simulink library "Miscellaneous"  (R2023a)
settings: Solver=ode45  StartTime=0.0  StopTime=10.0  RelTol=1e-3  EnableMultiTasking=on
libraries: simulink x4
(part 2 of 2)

== matlab function Miscellaneous/Merge2_Simulated/Merge_Simulated1 ==
  data: DataOut output Bus: BUS_UINT16_T; Data_1 input Bus: BUS_UINT16_T; Data_0 input Bus: BUS_UINT16_T
function DataOut = Or2(Data_1, Data_0)
    DataOut.b15 = Data_1.b15 || Data_0.b15;
    DataOut.b14 = Data_1.b14 || Data_0.b14;
    DataOut.b13 = Data_1.b13 || Data_0.b13;
    DataOut.b12 = Data_1.b12 || Data_0.b12;
    DataOut.b11 = Data_1.b11 || Data_0.b11;
    DataOut.b10 = Data_1.b10 || Data_0.b10;
    DataOut.b09 = Data_1.b09 || Data_0.b09;
    DataOut.b08 = Data_1.b08 || Data_0.b08;
    DataOut.b07 = Data_1.b07 || Data_0.b07;
    DataOut.b06 = Data_1.b06 || Data_0.b06;
    DataOut.b05 = Data_1.b05 || Data_0.b05;
    DataOut.b04 = Data_1.b04 || Data_0.b04;
    DataOut.b03 = Data_1.b03 || Data_0.b03;
    DataOut.b02 = Data_1.b02 || Data_0.b02;
    DataOut.b01 = Data_1.b01 || Data_0.b01;
    DataOut.b00 = Data_1.b00 || Data_0.b00;
end

== matlab function Miscellaneous/Merge16_Simulated ==
  data: Data_15 input Bus: BUS_UINT16_T; Data_14 input Bus: BUS_UINT16_T; Data_13 input Bus: BUS_UINT16_T size=1; Data_12 input Bus: BUS_UINT16_T; Data_11 input Bus: BUS_UINT16_T; Data_10 input Bus: BUS_UINT16_T; Data_09 input Bus: BUS_UINT16_T; Data_08 input Bus: BUS_UINT16_T; Data_07 input Bus: BUS_UINT16_T; Data_06 input Bus: BUS_UINT16_T; Data_05 input Bus: BUS_UINT16_T; Data_04 input Bus: BUS_UINT16_T; DataOut output Bus: BUS_UINT16_T; Data_03 input Bus: BUS_UINT16_T; Data_02 input Bus: BUS_UINT16_T; Data_01 input Bus: BUS_UINT16_T; Data_00 input Bus: BUS_UINT16_T
function DataOut = Or16(Data_15, Data_14, Data_13, Data_12, Data_11, Data_10, Data_09, Data_08, Data_07, Data_06, Data_05, Data_04, Data_03, Data_02, Data_01, Data_00)
    DataOut.b15 = Data_15.b15 || Data_14.b15 || Data_13.b15 || Data_12.b15 || Data_11.b15 || Data_10.b15 || Data_09.b15 || Data_08.b15 || Data_07.b15 || Data_06.b15 || Data_05.b15 || Data_04.b15 || Data_03.b15 || Data_02.b15 || Data_01.b15 || Data_00.b15;
    DataOut.b14 = Data_15.b14 || Data_14.b14 || Data_13.b14 || Data_12.b14 || Data_11.b14 || Data_10.b14 || Data_09.b14 || Data_08.b14 || Data_07.b14 || Data_06.b14 || Data_05.b14 || Data_04.b14 || Data_03.b14 || Data_02.b14 || Data_01.b14 || Data_00.b14;
    DataOut.b13 = Data_15.b13 || Data_14.b13 || Data_13.b13 || Data_12.b13 || Data_11.b13 || Data_10.b13 || Data_09.b13 || Data_08.b13 || Data_07.b13 || Data_06.b13 || Data_05.b13 || Data_04.b13 || Data_03.b13 || Data_02.b13 || Data_01.b13 || Data_00.b13;
    DataOut.b12 = Data_15.b12 || Data_14.b12 || Data_13.b12 || Data_12.b12 || Data_11.b12 || Data_10.b12 || Data_09.b12 || Data_08.b12 || Data_07.b12 || Data_06.b12 || Data_05.b12 || Data_04.b12 || Data_03.b12 || Data_02.b12 || Data_01.b12 || Data_00.b12;
    DataOut.b11 = Data_15.b11 || Data_14.b11 || Data_13.b11 || Data_12.b11 || Data_11.b11 || Data_10.b11 || Data_09.b11 || Data_08.b11 || Data_07.b11 || Data_06.b11 || Data_05.b11 || Data_04.b11 || Data_03.b11 || Data_02.b11 || Data_01.b11 || Data_00.b11;
    DataOut.b10 = Data_15.b10 || Data_14.b10 || Data_13.b10 || Data_12.b10 || Data_11.b10 || Data_10.b10 || Data_09.b10 || Data_08.b10 || Data_07.b10 || Data_06.b10 || Data_05.b10 || Data_04.b10 || Data_03.b10 || Data_02.b10 || Data_01.b10 || Data_00.b10;
    DataOut.b09 = Data_15.b09 || Data_14.b09 || Data_13.b09 || Data_12.b09 || Data_11.b09 || Data_10.b09 || Data_09.b09 || Data_08.b09 || Data_07.b09 || Data_06.b09 || Data_05.b09 || Data_04.b09 || Data_03.b09 || Data_02.b09 || Data_01.b09 || Data_00.b09;
    DataOut.b08 = Data_15.b08 || Data_14.b08 || Data_13.b08 || Data_12.b08 || Data_11.b08 || Data_10.b08 || Data_09.b08 || Data_08.b08 || Data_07.b08 || Data_06.b08 || Data_05.b08 || Data_04.b08 || Data_03.b08 || Data_02.b08 || Data_01.b08 || Data_00.b08;
    DataOut.b07 = Data_15.b07 || Data_14.b07 || Data_13.b07 || Data_12.b07 || Data_11.b07 || Data_10.b07 || Data_09.b07 || Data_08.b07 || Data_07.b07 || Data_06.b07 || Data_05.b07 || Data_04.b07 || Data_03.b07 || Data_02.b07 || Data_01.b07 || Data_00.b07;
    DataOut.b06 = Data_15.b06 || Data_14.b06 || Data_13.b06 || Data_12.b06 || Data_11.b06 || Data_10.b06 || Data_09.b06 || Data_08.b06 || Data_07.b06 || Data_06.b06 || Data_05.b06 || Data_04.b06 || Data_03.b06 || Data_02.b06 || Data_01.b06 || Data_00.b06;
    DataOut.b05 = Data_15.b05 || Data_14.b05 || Data_13.b05 || Data_12.b05 || Data_11.b05 || Data_10.b05 || Data_09.b05 || Data_08.b05 || Data_07.b05 || Data_06.b05 || Data_05.b05 || Data_04.b05 || Data_03.b05 || Data_02.b05 || Data_01.b05 || Data_00.b05;
    DataOut.b04 = Data_15.b04 || Data_14.b04 || Data_13.b04 || Data_12.b04 || Data_11.b04 || Data_10.b04 || Data_09.b04 || Data_08.b04 || Data_07.b04 || Data_06.b04 || Data_05.b04 || Data_04.b04 || Data_03.b04 || Data_02.b04 || Data_01.b04 || Data_00.b04;
    DataOut.b03 = Data_15.b03 || Data_14.b03 || Data_13.b03 || Data_12.b03 || Data_11.b03 || Data_10.b03 || Data_09.b03 || Data_08.b03 || Data_07.b03 || Data_06.b03 || Data_05.b03 || Data_04.b03 || Data_03.b03 || Data_02.b03 || Data_01.b03 || Data_00.b03;
    DataOut.b02 = Data_15.b02 || Data_14.b02 || Data_13.b02 || Data_12.b02 || Data_11.b02 || Data_10.b02 || Data_09.b02 || Data_08.b02 || Data_07.b02 || Data_06.b02 || Data_05.b02 || Data_04.b02 || Data_03.b02 || Data_02.b02 || Data_01.b02 || Data_00.b02;
    DataOut.b01 = Data_15.b01 || Data_14.b01 || Data_13.b01 || Data_12.b01 || Data_11.b01 || Data_10.b01 || Data_09.b01 || Data_08.b01 || Data_07.b01 || Data_06.b01 || Data_05.b01 || Data_04.b01 || Data_03.b01 || Data_02.b01 || Data_01.b01 || Data_00.b01;
    DataOut.b00 = Data_15.b00 || Data_14.b00 || Data_13.b00 || Data_12.b00 || Data_11.b00 || Data_10.b00 || Data_09.b00 || Data_08.b00 || Data_07.b00 || Data_06.b00 || Data_05.b00 || Data_04.b00 || Data_03.b00 || Data_02.b00 || Data_01.b00 || Data_00.b00;
end

== matlab function Miscellaneous/Merge8_Simulated ==
  data: Data_07 input Bus: BUS_UINT16_T; Data_06 input Bus: BUS_UINT16_T; Data_05 input Bus: BUS_UINT16_T; Data_04 input Bus: BUS_UINT16_T; DataOut output Bus: BUS_UINT16_T; Data_03 input Bus: BUS_UINT16_T; Data_02 input Bus: BUS_UINT16_T; Data_01 input Bus: BUS_UINT16_T; Data_00 input Bus: BUS_UINT16_T
function DataOut = Or8(Data_07, Data_06, Data_05, Data_04, Data_03, Data_02, Data_01, Data_00)
    DataOut.b15 = Data_07.b15 || Data_06.b15 || Data_05.b15 || Data_04.b15 || Data_03.b15 || Data_02.b15 || Data_01.b15 || Data_00.b15;
    DataOut.b14 = Data_07.b14 || Data_06.b14 || Data_05.b14 || Data_04.b14 || Data_03.b14 || Data_02.b14 || Data_01.b14 || Data_00.b14;
    DataOut.b13 = Data_07.b13 || Data_06.b13 || Data_05.b13 || Data_04.b13 || Data_03.b13 || Data_02.b13 || Data_01.b13 || Data_00.b13;
    DataOut.b12 = Data_07.b12 || Data_06.b12 || Data_05.b12 || Data_04.b12 || Data_03.b12 || Data_02.b12 || Data_01.b12 || Data_00.b12;
    DataOut.b11 = Data_07.b11 || Data_06.b11 || Data_05.b11 || Data_04.b11 || Data_03.b11 || Data_02.b11 || Data_01.b11 || Data_00.b11;
    DataOut.b10 = Data_07.b10 || Data_06.b10 || Data_05.b10 || Data_04.b10 || Data_03.b10 || Data_02.b10 || Data_01.b10 || Data_00.b10;
    DataOut.b09 = Data_07.b09 || Data_06.b09 || Data_05.b09 || Data_04.b09 || Data_03.b09 || Data_02.b09 || Data_01.b09 || Data_00.b09;
    DataOut.b08 = Data_07.b08 || Data_06.b08 || Data_05.b08 || Data_04.b08 || Data_03.b08 || Data_02.b08 || Data_01.b08 || Data_00.b08;
    DataOut.b07 = Data_07.b07 || Data_06.b07 || Data_05.b07 || Data_04.b07 || Data_03.b07 || Data_02.b07 || Data_01.b07 || Data_00.b07;
    DataOut.b06 = Data_07.b06 || Data_06.b06 || Data_05.b06 || Data_04.b06 || Data_03.b06 || Data_02.b06 || Data_01.b06 || Data_00.b06;
    DataOut.b05 = Data_07.b05 || Data_06.b05 || Data_05.b05 || Data_04.b05 || Data_03.b05 || Data_02.b05 || Data_01.b05 || Data_00.b05;
    DataOut.b04 = Data_07.b04 || Data_06.b04 || Data_05.b04 || Data_04.b04 || Data_03.b04 || Data_02.b04 || Data_01.b04 || Data_00.b04;
    DataOut.b03 = Data_07.b03 || Data_06.b03 || Data_05.b03 || Data_04.b03 || Data_03.b03 || Data_02.b03 || Data_01.b03 || Data_00.b03;
    DataOut.b02 = Data_07.b02 || Data_06.b02 || Data_05.b02 || Data_04.b02 || Data_03.b02 || Data_02.b02 || Data_01.b02 || Data_00.b02;
    DataOut.b01 = Data_07.b01 || Data_06.b01 || Data_05.b01 || Data_04.b01 || Data_03.b01 || Data_02.b01 || Data_01.b01 || Data_00.b01;
    DataOut.b00 = Data_07.b00 || Data_06.b00 || Data_05.b00 || Data_04.b00 || Data_03.b00 || Data_02.b00 || Data_01.b00 || Data_00.b00;
end

== matlab function Miscellaneous/Merge32_Simulated ==
  data: Data_31 input Bus: BUS_UINT16_T; Data_30 input Bus: BUS_UINT16_T; Data_29 input Bus: BUS_UINT16_T; Data_28 input Bus: BUS_UINT16_T; Data_27 input Bus: BUS_UINT16_T; Data_26 input Bus: BUS_UINT16_T; Data_25 input Bus: BUS_UINT16_T; Data_24 input Bus: BUS_UINT16_T; Data_23 input Bus: BUS_UINT16_T; Data_22 input Bus: BUS_UINT16_T; Data_21 input Bus: BUS_UINT16_T; Data_20 input Bus: BUS_UINT16_T; Data_19 input Bus: BUS_UINT16_T; Data_18 input Bus: BUS_UINT16_T; Data_17 input Bus: BUS_UINT16_T; Data_16 input Bus: BUS_UINT16_T; Data_15 input Bus: BUS_UINT16_T; Data_14 input Bus: BUS_UINT16_T; Data_13 input Bus: BUS_UINT16_T size=1; Data_12 input Bus: BUS_UINT16_T; Data_11 input Bus: BUS_UINT16_T; Data_10 input Bus: BUS_UINT16_T; Data_09 input Bus: BUS_UINT16_T; Data_08 input Bus: BUS_UINT16_T; Data_07 input Bus: BUS_UINT16_T; Data_06 input Bus: BUS_UINT16_T; Data_05 input Bus: BUS_UINT16_T; Data_04 input Bus: BUS_UINT16_T; DataOut output Bus: BUS_UINT16_T; Data_03 input Bus: BUS_UINT16_T; Data_02 input Bus: BUS_UINT16_T; Data_01 input Bus: BUS_UINT16_T; Data_00 input Bus: BUS_UINT16_T
function DataOut = Or32(Data_31, Data_30, Data_29, Data_28, Data_27, Data_26, Data_25, Data_24, Data_23, Data_22, Data_21, Data_20, Data_19, Data_18, Data_17, Data_16, Data_15, Data_14, Data_13, Data_12, Data_11, Data_10, Data_09, Data_08, Data_07, Data_06, Data_05, Data_04, Data_03, Data_02, Data_01, Data_00)
    DataOut.b15 = Data_31.b15 || Data_30.b15 || Data_29.b15 || Data_28.b15 || Data_27.b15 || Data_26.b15 || Data_25.b15 || Data_24.b15 || Data_23.b15 || Data_22.b15 || Data_21.b15 || Data_20.b15 || Data_19.b15 || Data_18.b15 || Data_17.b15 || Data_16.b15 || Data_15.b15 || Data_14.b15 || Data_13.b15 || Data_12.b15 || Data_11.b15 || Data_10.b15 || Data_09.b15 || Data_08.b15 || Data_07.b15 || Data_06.b15 || Data_05.b15 || Data_04.b15 || Data_03.b15 || Data_02.b15 || Data_01.b15 || Data_00.b15;
    DataOut.b14 = Data_31.b14 || Data_30.b14 || Data_29.b14 || Data_28.b14 || Data_27.b14 || Data_26.b14 || Data_25.b14 || Data_24.b14 || Data_23.b14 || Data_22.b14 || Data_21.b14 || Data_20.b14 || Data_19.b14 || Data_18.b14 || Data_17.b14 || Data_16.b14 || Data_15.b14 || Data_14.b14 || Data_13.b14 || Data_12.b14 || Data_11.b14 || Data_10.b14 || Data_09.b14 || Data_08.b14 || Data_07.b14 || Data_06.b14 || Data_05.b14 || Data_04.b14 || Data_03.b14 || Data_02.b14 || Data_01.b14 || Data_00.b14;
    DataOut.b13 = Data_31.b13 || Data_30.b13 || Data_29.b13 || Data_28.b13 || Data_27.b13 || Data_26.b13 || Data_25.b13 || Data_24.b13 || Data_23.b13 || Data_22.b13 || Data_21.b13 || Data_20.b13 || Data_19.b13 || Data_18.b13 || Data_17.b13 || Data_16.b13 || Data_15.b13 || Data_14.b13 || Data_13.b13 || Data_12.b13 || Data_11.b13 || Data_10.b13 || Data_09.b13 || Data_08.b13 || Data_07.b13 || Data_06.b13 || Data_05.b13 || Data_04.b13 || Data_03.b13 || Data_02.b13 || Data_01.b13 || Data_00.b13;
    DataOut.b12 = Data_31.b12 || Data_30.b12 || Data_29.b12 || Data_28.b12 || Data_27.b12 || Data_26.b12 || Data_25.b12 || Data_24.b12 || Data_23.b12 || Data_22.b12 || Data_21.b12 || Data_20.b12 || Data_19.b12 || Data_18.b12 || Data_17.b12 || Data_16.b12 || Data_15.b12 || Data_14.b12 || Data_13.b12 || Data_12.b12 || Data_11.b12 || Data_10.b12 || Data_09.b12 || Data_08.b12 || Data_07.b12 || Data_06.b12 || Data_05.b12 || Data_04.b12 || Data_03.b12 || Data_02.b12 || Data_01.b12 || Data_00.b12;
    DataOut.b11 = Data_31.b11 || Data_30.b11 || Data_29.b11 || Data_28.b11 || Data_27.b11 || Data_26.b11 || Data_25.b11 || Data_24.b11 || Data_23.b11 || Data_22.b11 || Data_21.b11 || Data_20.b11 || Data_19.b11 || Data_18.b11 || Data_17.b11 || Data_16.b11 || Data_15.b11 || Data_14.b11 || Data_13.b11 || Data_12.b11 || Data_11.b11 || Data_10.b11 || Data_09.b11 || Data_08.b11 || Data_07.b11 || Data_06.b11 || Data_05.b11 || Data_04.b11 || Data_03.b11 || Data_02.b11 || Data_01.b11 || Data_00.b11;
    DataOut.b10 = Data_31.b10 || Data_30.b10 || Data_29.b10 || Data_28.b10 || Data_27.b10 || Data_26.b10 || Data_25.b10 || Data_24.b10 || Data_23.b10 || Data_22.b10 || Data_21.b10 || Data_20.b10 || Data_19.b10 || Data_18.b10 || Data_17.b10 || Data_16.b10 || Data_15.b10 || Data_14.b10 || Data_13.b10 || Data_12.b10 || Data_11.b10 || Data_10.b10 || Data_09.b10 || Data_08.b10 || Data_07.b10 || Data_06.b10 || Data_05.b10 || Data_04.b10 || Data_03.b10 || Data_02.b10 || Data_01.b10 || Data_00.b10;
    DataOut.b09 = Data_31.b09 || Data_30.b09 || Data_29.b09 || Data_28.b09 || Data_27.b09 || Data_26.b09 || Data_25.b09 || Data_24.b09 || Data_23.b09 || Data_22.b09 || Data_21.b09 || Data_20.b09 || Data_19.b09 || Data_18.b09 || Data_17.b09 || Data_16.b09 || Data_15.b09 || Data_14.b09 || Data_13.b09 || Data_12.b09 || Data_11.b09 || Data_10.b09 || Data_09.b09 || Data_08.b09 || Data_07.b09 || Data_06.b09 || Data_05.b09 || Data_04.b09 || Data_03.b09 || Data_02.b09 || Data_01.b09 || Data_00.b09;
    DataOut.b08 = Data_31.b08 || Data_30.b08 || Data_29.b08 || Data_28.b08 || Data_27.b08 || Data_26.b08 || Data_25.b08 || Data_24.b08 || Data_23.b08 || Data_22.b08 || Data_21.b08 || Data_20.b08 || Data_19.b08 || Data_18.b08 || Data_17.b08 || Data_16.b08 || Data_15.b08 || Data_14.b08 || Data_13.b08 || Data_12.b08 || Data_11.b08 || Data_10.b08 || Data_09.b08 || Data_08.b08 || Data_07.b08 || Data_06.b08 || Data_05.b08 || Data_04.b08 || Data_03.b08 || Data_02.b08 || Data_01.b08 || Data_00.b08;
    DataOut.b07 = Data_31.b07 || Data_30.b07 || Data_29.b07 || Data_28.b07 || Data_27.b07 || Data_26.b07 || Data_25.b07 || Data_24.b07 || Data_23.b07 || Data_22.b07 || Data_21.b07 || Data_20.b07 || Data_19.b07 || Data_18.b07 || Data_17.b07 || Data_16.b07 || Data_15.b07 || Data_14.b07 || Data_13.b07 || Data_12.b07 || Data_11.b07 || Data_10.b07 || Data_09.b07 || Data_08.b07 || Data_07.b07 || Data_06.b07 || Data_05.b07 || Data_04.b07 || Data_03.b07 || Data_02.b07 || Data_01.b07 || Data_00.b07;
    DataOut.b06 = Data_31.b06 || Data_30.b06 || Data_29.b06 || Data_28.b06 || Data_27.b06 || Data_26.b06 || Data_25.b06 || Data_24.b06 || Data_23.b06 || Data_22.b06 || Data_21.b06 || Data_20.b06 || Data_19.b06 || Data_18.b06 || Data_17.b06 || Data_16.b06 || Data_15.b06 || Data_14.b06 || Data_13.b06 || Data_12.b06 || Data_11.b06 || Data_10.b06 || Data_09.b06 || Data_08.b06 || Data_07.b06 || Data_06.b06 || Data_05.b06 || Data_04.b06 || Data_03.b06 || Data_02.b06 || Data_01.b06 || Data_00.b06;
    DataOut.b05 = Data_31.b05 || Data_30.b05 || Data_29.b05 || Data_28.b05 || Data_27.b05 || Data_26.b05 || Data_25.b05 || Data_24.b05 || Data_23.b05 || Data_22.b05 || Data_21.b05 || Data_20.b05 || Data_19.b05 || Data_18.b05 || Data_17.b05 || Data_16.b05 || Data_15.b05 || Data_14.b05 || Data_13.b05 || Data_12.b05 || Data_11.b05 || Data_10.b05 || Data_09.b05 || Data_08.b05 || Data_07.b05 || Data_06.b05 || Data_05.b05 || Data_04.b05 || Data_03.b05 || Data_02.b05 || Data_01.b05 || Data_00.b05;
    DataOut.b04 = Data_31.b04 || Data_30.b04 || Data_29.b04 || Data_28.b04 || Data_27.b04 || Data_26.b04 || Data_25.b04 || Data_24.b04 || Data_23.b04 || Data_22.b04 || Data_21.b04 || Data_20.b04 || Data_19.b04 || Data_18.b04 || Data_17.b04 || Data_16.b04 || Data_15.b04 || Data_14.b04 || Data_13.b04 || Data_12.b04 || Data_11.b04 || Data_10.b04 || Data_09.b04 || Data_08.b04 || Data_07.b04 || Data_06.b04 || Data_05.b04 || Data_04.b04 || Data_03.b04 || Data_02.b04 || Data_01.b04 || Data_00.b04;
    DataOut.b03 = Data_31.b03 || Data_30.b03 || Data_29.b03 || Data_28.b03 || Data_27.b03 || Data_26.b03 || Data_25.b03 || Data_24.b03 || Data_23.b03 || Data_22.b03 || Data_21.b03 || Data_20.b03 || Data_19.b03 || Data_18.b03 || Data_17.b03 || Data_16.b03 || Data_15.b03 || Data_14.b03 || Data_13.b03 || Data_12.b03 || Data_11.b03 || Data_10.b03 || Data_09.b03 || Data_08.b03 || Data_07.b03 || Data_06.b03 || Data_05.b03 || Data_04.b03 || Data_03.b03 || Data_02.b03 || Data_01.b03 || Data_00.b03;
    DataOut.b02 = Data_31.b02 || Data_30.b02 || Data_29.b02 || Data_28.b02 || Data_27.b02 || Data_26.b02 || Data_25.b02 || Data_24.b02 || Data_23.b02 || Data_22.b02 || Data_21.b02 || Data_20.b02 || Data_19.b02 || Data_18.b02 || Data_17.b02 || Data_16.b02 || Data_15.b02 || Data_14.b02 || Data_13.b02 || Data_12.b02 || Data_11.b02 || Data_10.b02 || Data_09.b02 || Data_08.b02 || Data_07.b02 || Data_06.b02 || Data_05.b02 || Data_04.b02 || Data_03.b02 || Data_02.b02 || Data_01.b02 || Data_00.b02;
    DataOut.b01 = Data_31.b01 || Data_30.b01 || Data_29.b01 || Data_28.b01 || Data_27.b01 || Data_26.b01 || Data_25.b01 || Data_24.b01 || Data_23.b01 || Data_22.b01 || Data_21.b01 || Data_20.b01 || Data_19.b01 || Data_18.b01 || Data_17.b01 || Data_16.b01 || Data_15.b01 || Data_14.b01 || Data_13.b01 || Data_12.b01 || Data_11.b01 || Data_10.b01 || Data_09.b01 || Data_08.b01 || Data_07.b01 || Data_06.b01 || Data_05.b01 || Data_04.b01 || Data_03.b01 || Data_02.b01 || Data_01.b01 || Data_00.b01;
    DataOut.b00 = Data_31.b00 || Data_30.b00 || Data_29.b00 || Data_28.b00 || Data_27.b00 || Data_26.b00 || Data_25.b00 || Data_24.b00 || Data_23.b00 || Data_22.b00 || Data_21.b00 || Data_20.b00 || Data_19.b00 || Data_18.b00 || Data_17.b00 || Data_16.b00 || Data_15.b00 || Data_14.b00 || Data_13.b00 || Data_12.b00 || Data_11.b00 || Data_10.b00 || Data_09.b00 || Data_08.b00 || Data_07.b00 || Data_06.b00 || Data_05.b00 || Data_04.b00 || Data_03.b00 || Data_02.b00 || Data_01.b00 || Data_00.b00;
end
